simulink model "bloque_fuzzy"  (R2023a)
settings: Solver=VariableStepAuto  StartTime=0.0  StopTime=10.0  RelTol=1e-3
libraries: fuzblock x1
settings Model: Creator=mfran  LastModifiedBy=mfran

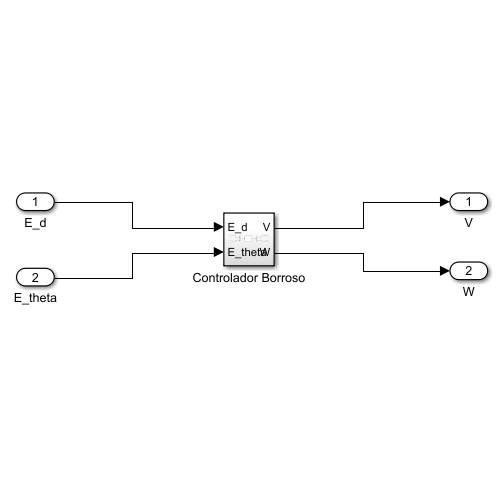
[thumbnail: Simulink's stored preview of the top-level diagram]
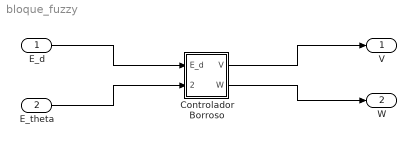
== system bloque_fuzzy ==
  E_d : Inport
  E_theta : Inport  Port=2
  Controlador Borroso : Subsystem
  V : Outport
  W : Outport  Port=2
  wires:
  E_d/1 -> Controlador Borroso/1(E_d)
  E_theta/1 -> Controlador Borroso/2(E_theta)
  Controlador Borroso/1(V) -> V/1
  Controlador Borroso/2(W) -> W/1

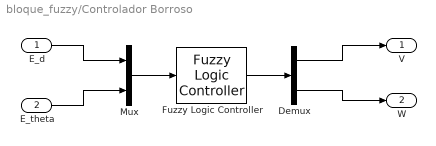
== system bloque_fuzzy/Controlador Borroso ==
  E_d : Inport
  E_theta : Inport  Port=2
  Demux : Demux  Outputs=2
  Fuzzy Logic Controller : fuzblock/Fuzzy Logic  Controller  FIS='version1.fis'  OutputSampleNumber=101  DataType=double  FuzzifiedInputs=off  RuleFiringStrengths=off  RuleOutputs=off  AggregatedOutputs=off  SimulateUsing=Interpreted execution  OutOfRangeInputValueMessage=warning  NoRuleFiredMessage=warning  EmptyOutputFuzzySetMessage=warning
  Mux : Mux  Inputs=2
  V : Outport
  W : Outport  Port=2
  wires:
  Demux/1 -> V/1
  Fuzzy Logic Controller/1 -> Demux/1
  Demux/2 -> W/1
  E_theta/1 -> Mux/2
  E_d/1 -> Mux/1
  Mux/1 -> Fuzzy Logic Controller/1
